simulink model "TASK_COUNTER"  (R2016a)
settings: Solver=FixedStepDiscrete  StartTime=0.0  StopTime=10.0  RelTol=1e-3
model workspace (MAT data in the model file):
  cs : Simulink.ConfigSet (value not decoded)
settings Model: Creator=LEGION  LastModifiedBy=LEGION

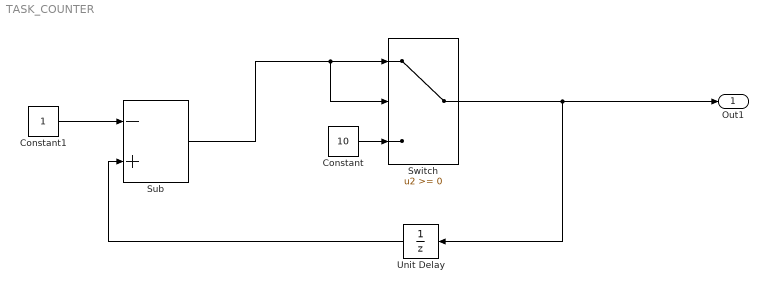
== system TASK_COUNTER ==
  Constant : Constant  Value=10
  Constant1 : Constant
  "Sub " : Sum  Inputs=-+
  Switch : Switch
  Unit Delay : UnitDelay  SampleTime=-1
  Out1 : Outport
  wires:
  Switch/1 -> Out1/1, Unit Delay/1
  Unit Delay/1 -> "Sub "/2
  Constant1/1 -> "Sub "/1
  "Sub "/1 -> Switch/2, Switch/1
  Constant/1 -> Switch/3
